simulink subsystem "quaternionMultiplication"  (R2025b)
settings: Solver=VariableStepAuto  StartTime=0.0  StopTime=10.0  RelTol=1e-3
model mask{quatMultType=Type 1, quatConv=q0, normQuat=Yes}
  mask prompts: quatMultType "Multiplication type"; quatConv "Scalar convention"; normQuat "Normalize quaternion"
libraries: matrix_library x2
settings Model: Creator=antoniohernandez-rodiciomateos  LastModifiedBy=antoniohernandez-rodiciomateos

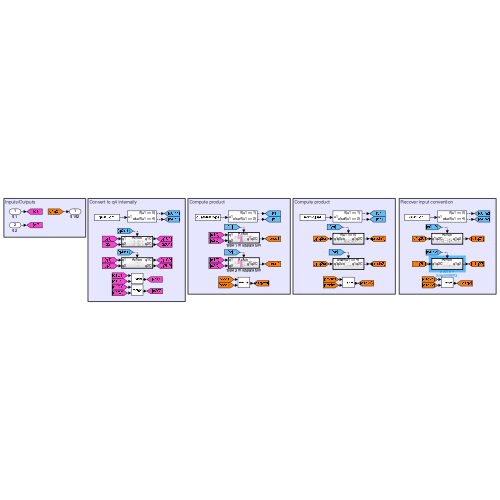
[thumbnail: Simulink's stored preview of the top-level diagram]
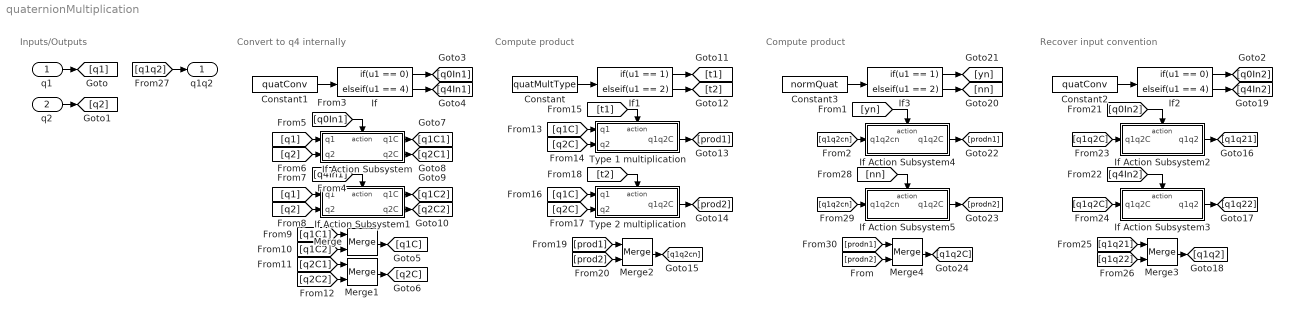
== system quaternionMultiplication ==
  note: Inputs/Outputs
  note: Convert to q4 internally
  note: Compute product
  note: Recover input convention
  note: Compute product
  q1 : Inport  OutDataTypeStr=double  PortDimensions=[4 1]
  q2 : Inport  Port=2  OutDataTypeStr=double  PortDimensions=[4 1]
  Constant : Constant  Value=quatMultType
  Constant1 : Constant  Value=quatConv
  Constant2 : Constant  Value=quatConv
  Constant3 : Constant  Value=normQuat
  If : If  IfExpression=u1 == 0  ElseIfExpressions=u1 == 4  ShowElse=off
  If Action Subsystem : Subsystem  TreatAsAtomicUnit=on
  If Action Subsystem1 : Subsystem  TreatAsAtomicUnit=on
  If Action Subsystem2 : Subsystem  TreatAsAtomicUnit=on
  If Action Subsystem3 : Subsystem  TreatAsAtomicUnit=on
  If Action Subsystem4 : Subsystem  TreatAsAtomicUnit=on
  If Action Subsystem5 : Subsystem  TreatAsAtomicUnit=on
  If1 : If  IfExpression=u1 == 1  ElseIfExpressions=u1 == 2  ShowElse=off
  If2 : If  IfExpression=u1 == 0  ElseIfExpressions=u1 == 4  ShowElse=off
  If3 : If  IfExpression=u1 == 1  ElseIfExpressions=u1 == 2  ShowElse=off
  Merge{,1..4} (5 alike) : Merge
  Type 1 multiplication : Subsystem  TreatAsAtomicUnit=on
  Type 2 multiplication : Subsystem  TreatAsAtomicUnit=on
  q1q2 : Outport  OutDataTypeStr=double  PortDimensions=[4 1]
  wires:
  q1/1 -> [q1]
  q2/1 -> [q2]
  [q1q2] -> q1q2/1
  Constant1/1 -> If/1
  If/1 -> [q0In1]
  If/2 -> [q4In1]
  [q0In1] -> If Action Subsystem/Action
  [q1] -> If Action Subsystem/1(q1)
  [q2] -> If Action Subsystem/2(q2)
  [q2] -> If Action Subsystem1/2(q2)
  [q1] -> If Action Subsystem1/1(q1)
  [q4In1] -> If Action Subsystem1/Action
  If Action Subsystem/1(q1C) -> [q1C1]
  If Action Subsystem/2(q2C) -> [q2C1]
  If Action Subsystem1/1(q1C) -> [q1C2]
  If Action Subsystem1/2(q2C) -> [q2C2]
  [q1C1] -> Merge/1
  [q1C2] -> Merge/2
  [q2C1] -> Merge1/1
  [q2C2] -> Merge1/2
  Merge/1 -> [q1C]
  Merge1/1 -> [q2C]
  If1/2 -> [t2]
  If1/1 -> [t1]
  Constant/1 -> If1/1
  [q2C] -> Type 1 multiplication/2(q2)
  [q1C] -> Type 1 multiplication/1(q1)
  [t1] -> Type 1 multiplication/Action
  Type 1 multiplication/1(q1q2C) -> [prod1]
  [t2] -> Type 2 multiplication/Action
  [q2C] -> Type 2 multiplication/2(q2)
  [q1C] -> Type 2 multiplication/1(q1)
  Type 2 multiplication/1(q1q2C) -> [prod2]
  [prod1] -> Merge2/1
  Merge2/1 -> [q1q2cn]
  [prod2] -> Merge2/2
  [q0In2] -> If Action Subsystem2/Action
  [q4In2] -> If Action Subsystem3/Action
  [q1q2C] -> If Action Subsystem2/1(q1q2C)
  [q1q2C] -> If Action Subsystem3/1(q1q2C)
  If Action Subsystem2/1(q1q2) -> [q1q21]
  If Action Subsystem3/1(q1q2) -> [q1q22]
  Merge3/1 -> [q1q2]
  [q1q22] -> Merge3/2
  [q1q21] -> Merge3/1
  Constant2/1 -> If2/1
  If2/1 -> [q0In2]
  If2/2 -> [q4In2]
  If3/1 -> [yn]
  Constant3/1 -> If3/1
  If3/2 -> [nn]
  [q1q2cn] -> If Action Subsystem4/1(q1q2cn)
  [yn] -> If Action Subsystem4/Action
  If Action Subsystem4/1(q1q2C) -> [prodn1]
  [nn] -> If Action Subsystem5/Action
  [q1q2cn] -> If Action Subsystem5/1(q1q2cn)
  If Action Subsystem5/1(q1q2C) -> [prodn2]
  [prodn1] -> Merge4/1
  [prodn2] -> Merge4/2
  Merge4/1 -> [q1q2C]

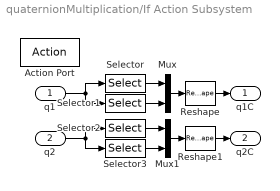
== system quaternionMultiplication/If Action Subsystem ==
  q1 : Inport  OutDataTypeStr=double  PortDimensions=[4 1]
  q2 : Inport  Port=2  OutDataTypeStr=double  PortDimensions=[4 1]
  Action Port : ActionPort
  Mux : Mux  Inputs=2
  Mux1 : Mux  Inputs=2
  Reshape : Reshape  OutputDimensionality=Column vector (2-D)
  Reshape1 : Reshape  OutputDimensionality=Column vector (2-D)
  Selector : Selector  InputPortWidth=4  IndexOptions=Index vector (dialog)  Indices=[2 3 4]  OutputSizes=1
  Selector1 : Selector  InputPortWidth=4  IndexOptions=Index vector (dialog)  Indices=[1]  OutputSizes=1
  Selector2 : Selector  InputPortWidth=4  IndexOptions=Index vector (dialog)  Indices=[2 3 4]  OutputSizes=1
  Selector3 : Selector  InputPortWidth=4  IndexOptions=Index vector (dialog)  Indices=[1]  OutputSizes=1
  q1C : Outport  OutDataTypeStr=double  PortDimensions=[4 1]
  q2C : Outport  Port=2  OutDataTypeStr=double  PortDimensions=[4 1]
  wires:
  q1/1 -> Selector1/1, Selector/1
  Selector1/1 -> Mux/2
  Selector/1 -> Mux/1
  Mux/1 -> Reshape/1
  Reshape/1 -> q1C/1
  Reshape1/1 -> q2C/1
  q2/1 -> Selector3/1, Selector2/1
  Selector2/1 -> Mux1/1
  Selector3/1 -> Mux1/2
  Mux1/1 -> Reshape1/1

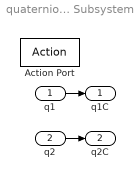
== system quaternionMultiplication/If Action Subsystem1 ==
  q1 : Inport  OutDataTypeStr=double  PortDimensions=[4 1]
  q2 : Inport  Port=2  OutDataTypeStr=double  PortDimensions=[4 1]
  Action Port : ActionPort
  q1C : Outport  OutDataTypeStr=double  PortDimensions=[4 1]
  q2C : Outport  Port=2  OutDataTypeStr=double  PortDimensions=[4 1]
  wires:
  q1/1 -> q1C/1
  q2/1 -> q2C/1

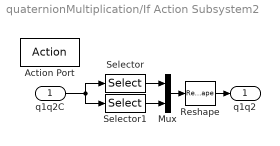
== system quaternionMultiplication/If Action Subsystem2 ==
  q1q2C : Inport  OutDataTypeStr=double  PortDimensions=[4 1]
  Action Port : ActionPort
  Mux : Mux  Inputs=2
  Reshape : Reshape  OutputDimensionality=Column vector (2-D)
  Selector : Selector  InputPortWidth=4  IndexOptions=Index vector (dialog)  Indices=[4]  OutputSizes=1
  Selector1 : Selector  InputPortWidth=4  IndexOptions=Index vector (dialog)  Indices=[1 2 3]  OutputSizes=1
  q1q2 : Outport  OutDataTypeStr=double  PortDimensions=[4 1]
  wires:
  q1q2C/1 -> Selector1/1, Selector/1
  Selector1/1 -> Mux/2
  Selector/1 -> Mux/1
  Mux/1 -> Reshape/1
  Reshape/1 -> q1q2/1

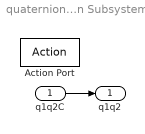
== system quaternionMultiplication/If Action Subsystem3 ==
  q1q2C : Inport  OutDataTypeStr=double  PortDimensions=[4 1]
  Action Port : ActionPort
  q1q2 : Outport  OutDataTypeStr=double  PortDimensions=[4 1]
  wires:
  q1q2C/1 -> q1q2/1

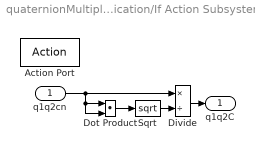
== system quaternionMultiplication/If Action Subsystem4 ==
  q1q2cn : Inport  OutDataTypeStr=double  PortDimensions=[4 1]
  Action Port : ActionPort  ActionPortLabel=if(u1 == 0)
  Divide : Product  Inputs=*/
  Dot Product : DotProduct  OutDataTypeStr=Inherit: Inherit via internal rule
  Sqrt : Sqrt
  q1q2C : Outport  OutDataTypeStr=double  PortDimensions=[4 1]
  wires:
  Divide/1 -> q1q2C/1
  q1q2cn/1 -> Divide/1, Dot Product/2, Dot Product/1
  Dot Product/1 -> Sqrt/1
  Sqrt/1 -> Divide/2

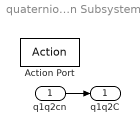
== system quaternionMultiplication/If Action Subsystem5 ==
  q1q2cn : Inport  OutDataTypeStr=double  PortDimensions=[4 1]
  Action Port : ActionPort  ActionPortLabel=elseif(u1 == 4)
  q1q2C : Outport  OutDataTypeStr=double  PortDimensions=[4 1]
  wires:
  q1q2cn/1 -> q1q2C/1

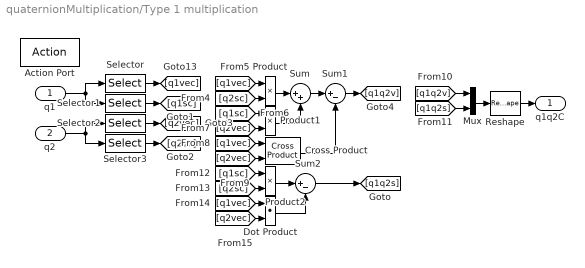
== system quaternionMultiplication/Type 1 multiplication ==
  q1 : Inport  OutDataTypeStr=double  PortDimensions=[4 1]
  q2 : Inport  Port=2  OutDataTypeStr=double  PortDimensions=[4 1]
  Action Port : ActionPort
  Cross Product : matrix_library/Cross Product
  Dot Product : DotProduct  OutDataTypeStr=Inherit: Inherit via internal rule
  Mux : Mux  Inputs=2
  Product : Product
  Product1 : Product
  Product2 : Product
  Reshape : Reshape  OutputDimensionality=Column vector (2-D)
  Selector : Selector  InputPortWidth=4  IndexOptions=Index vector (dialog)  Indices=[1 2 3]  OutputSizes=1
  Selector1 : Selector  InputPortWidth=4  IndexOptions=Index vector (dialog)  Indices=[4]  OutputSizes=1
  Selector2 : Selector  InputPortWidth=4  IndexOptions=Index vector (dialog)  Indices=[1 2 3]  OutputSizes=1
  Selector3 : Selector  InputPortWidth=4  IndexOptions=Index vector (dialog)  Indices=[4]  OutputSizes=1
  Sum : Sum  Inputs=|++
  Sum1 : Sum  Inputs=|+-
  Sum2 : Sum  Inputs=|+-
  q1q2C : Outport  OutDataTypeStr=double  PortDimensions=[4 1]
  wires:
  q1/1 -> Selector1/1, Selector/1
  Selector1/1 -> [q1sc]
  Selector/1 -> [q1vec]
  Reshape/1 -> q1q2C/1
  q2/1 -> Selector3/1, Selector2/1
  Selector2/1 -> [q2vec]
  Selector3/1 -> [q2sc]
  Mux/1 -> Reshape/1
  [q2sc] -> Product/2
  [q1vec] -> Product/1
  Product/1 -> Sum/1
  [q1sc] -> Product1/1
  [q2vec] -> Product1/2
  Product1/1 -> Sum/2
  Sum/1 -> Sum1/1
  [q1vec] -> Cross Product/1
  [q2vec] -> Cross Product/2
  Cross Product/1 -> Sum1/2
  Sum1/1 -> [q1q2v]
  [q1q2v] -> Mux/1
  [q1q2s] -> Mux/2
  [q1sc] -> Product2/1
  [q2sc] -> Product2/2
  Product2/1 -> Sum2/1
  [q1vec] -> Dot Product/1
  [q2vec] -> Dot Product/2
  Dot Product/1 -> Sum2/2
  Sum2/1 -> [q1q2s]

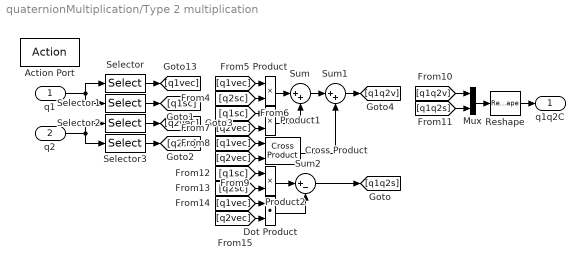
== system quaternionMultiplication/Type 2 multiplication ==
  q1 : Inport  OutDataTypeStr=double  PortDimensions=[4 1]
  q2 : Inport  Port=2  OutDataTypeStr=double  PortDimensions=[4 1]
  Action Port : ActionPort
  Cross Product : matrix_library/Cross Product
  Dot Product : DotProduct  OutDataTypeStr=Inherit: Inherit via internal rule
  Mux : Mux  Inputs=2
  Product : Product
  Product1 : Product
  Product2 : Product
  Reshape : Reshape  OutputDimensionality=Column vector (2-D)
  Selector : Selector  InputPortWidth=4  IndexOptions=Index vector (dialog)  Indices=[1 2 3]  OutputSizes=1
  Selector1 : Selector  InputPortWidth=4  IndexOptions=Index vector (dialog)  Indices=[4]  OutputSizes=1
  Selector2 : Selector  InputPortWidth=4  IndexOptions=Index vector (dialog)  Indices=[1 2 3]  OutputSizes=1
  Selector3 : Selector  InputPortWidth=4  IndexOptions=Index vector (dialog)  Indices=[4]  OutputSizes=1
  Sum : Sum  Inputs=|++
  Sum1 : Sum  Inputs=|++
  Sum2 : Sum  Inputs=|+-
  q1q2C : Outport  OutDataTypeStr=double  PortDimensions=[4 1]
  wires:
  q1/1 -> Selector1/1, Selector/1
  Selector1/1 -> [q1sc]
  Selector/1 -> [q1vec]
  Reshape/1 -> q1q2C/1
  q2/1 -> Selector3/1, Selector2/1
  Selector2/1 -> [q2vec]
  Selector3/1 -> [q2sc]
  Mux/1 -> Reshape/1
  [q2sc] -> Product/2
  [q1vec] -> Product/1
  Product/1 -> Sum/1
  [q1sc] -> Product1/1
  [q2vec] -> Product1/2
  Product1/1 -> Sum/2
  Sum/1 -> Sum1/1
  [q1vec] -> Cross Product/1
  [q2vec] -> Cross Product/2
  Cross Product/1 -> Sum1/2
  Sum1/1 -> [q1q2v]
  [q1q2v] -> Mux/1
  [q1q2s] -> Mux/2
  [q1sc] -> Product2/1
  [q2sc] -> Product2/2
  Product2/1 -> Sum2/1
  [q1vec] -> Dot Product/1
  [q2vec] -> Dot Product/2
  Dot Product/1 -> Sum2/2
  Sum2/1 -> [q1q2s]
